simulink model "hamiltonian_record"  (R2012b)
settings: Solver=ode3  StartTime=0.0  StopTime=10  FixedStep=0.001  RelTol=1e-3
settings Model: ExtModeTrigDuration=5000  Creator=yiwei.liu  LastModifiedBy=yiwei.liu
settings SolverCC: PositivePriorityOrder=on
settings RTWCC: SystemTargetFile=quarc_win64.tlc  TemplateMakefile=quarc_default_tmf  Description=QUARC Win64 Target  ProcessScript=quarc_win64_make_rtw_hook
settings STFCustomTargetCC: TargetPreCompLibLocation=C:\PROGRA~3\QUARC\lib\2012b\win64\release  CodeReplacementLibrary=ANSI_C  GeneratePreprocessorConditionals=Disable all  CombineOutputUpdateFcns=on  GRTInterface=off  SystemTargetFile=quarc_win64.tlc
settings GRTTargetCC: TargetPreCompLibLocation=C:\PROGRA~3\QUARC\lib\2012b\win64\release  ParMdlRefBuildCompliant=off  CompOptLevelCompliant=off  ConcurrentExecutionCompliant=off  MatFileLogging=off  ExtMode=on  ExtModeMexFile=quarc_comm

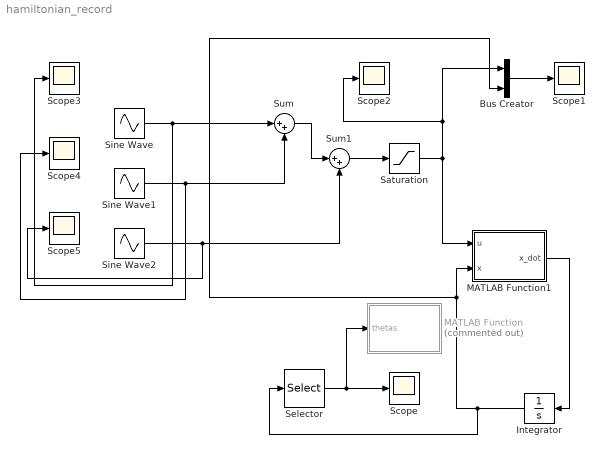
== system hamiltonian_record ==
  Bus Creator : BusCreator  Inputs=2
  Integrator : Integrator  InitialCondition=[0;0;pi;0]
  MATLAB Function : MATLAB Function  Commented=on  TreatAsAtomicUnit=on
  MATLAB Function1 : MATLAB Function  TreatAsAtomicUnit=on
  Saturation : Saturate  UpperLimit=10  LowerLimit=-10
  Scope{,1..5} (6 alike) : Scope
      Scope settings: YMin=-0.25  YMax=5.25
      Scope1 settings: ShowLegends=on  YMin=-7  YMax=8  SaveName=sim  MaxDataPoints=10000
      Scope2 settings: ShowLegends=on  YMin=-7.5  YMax=10  SaveName=rbd1  MaxDataPoints=10000
      Scope3 settings: ShowLegends=on  SaveName=rbd2  MaxDataPoints=10000
      Scope4 settings: ShowLegends=on  SaveName=rbd3  MaxDataPoints=10000
      Scope5 settings: ShowLegends=on  YMin=-3  YMax=7  SaveName=rbd4  MaxDataPoints=10000
  Selector : Selector  InputPortWidth=4  IndexOptions=Index vector (dialog)  Indices=[1 3]  OutputSizes=1
  Sine Wave : Sin  Amplitude=5  Frequency=5  Phase=0.8  SampleTime=0
  Sine Wave1 : Sin  Amplitude=5  Frequency=10  Phase=1.2  SampleTime=0
  Sine Wave2 : Sin  Amplitude=5  Frequency=20  Phase=0.4  SampleTime=0
  Sum : Sum  Inputs=|++
  Sum1 : Sum  Inputs=|++
  wires:
  MATLAB Function1/1(x_dot) -> Integrator/1
  Integrator/1 -> Bus Creator/2, MATLAB Function1/2(x), Selector/1
  Selector/1 -> MATLAB Function/1(thetas), Scope/1
  Sum/1 -> Sum1/1
  Bus Creator/1 -> Scope1/1
  Sine Wave2/1 -> Scope5/1, Sum1/2
  Sine Wave/1 -> Scope3/1, Sum/1
  Sine Wave1/1 -> Scope4/1, Sum/2
  Saturation/1 -> MATLAB Function1/1(u), Scope2/1, Bus Creator/1
  Sum1/1 -> Saturation/1

== matlab function hamiltonian_record/MATLAB Function ==
  data: thetas input
function  fcn(thetas)
%#codegen
A=[0 0 0 0 0];
B=[0 0 6 6 8];
C=[0 -1 -1 0 0];
D=[1 1 1 1 1];

A2=[0 0];
B2=[0 12];
C2=[0 0];
D2=[1 1];
L1=6;

L2=2;
%First Link

    theta1=thetas(1);
    theta2=thetas(2);
    newpoints=trans(theta1,A,B,C,D);
    p= (newpoints(1:1,1:5));

    q= (newpoints(2:2,1:5));

    r= (newpoints(3:3,1:5));
   % Second Link

    new2=trans2(theta2,L1,L2,A2,B2,C2,D2);
    %Frame 1 to frame 0
    x2= new2(1:1,1:2);
    y2= new2(2:2,1:2);
    z2= new2(3:3,1:2);

    new3 = trans(theta1,x2,y2,z2,D2);
    %ABC values of Link 2 in frame 0
    p2= (new3(1:1,1:2));

    q2= (new3(2:2,1:2));

    r2= (new3(3:3,1:2));
   
%     hold on;

    plot3(p,q,r,'-b*',p2,q2,r2,'-g*');
    axis([-15,15,-15,15,-15,15]);
    grid on;
end

== matlab function hamiltonian_record/MATLAB Function1 ==
  data: u input; x_dot output; x input
function x_dot = fcn(u,x)
%#codegen
 
theta1= 0.0304;
theta2= 0.0184;
theta3= 0.0184;
theta4= 0.0921;
theta5= 0.6101;
theta6= 0.0097;

q1 = x(1);
q1_dot = x(2);
q2 = x(3);
q2_dot = x(4);
 
v = [u ; 0];
A = [theta1+theta2*(sin(q2)^2), theta3*cos(q2) ; theta3*cos(q2), theta2];
B = [2*theta2*sin(q2)*cos(q2)*q2_dot, (-1)*theta3*sin(q2)*q2_dot; (-1)*theta2*sin(q2)*cos(q2)*q1_dot,  0];
C = [theta5*q1_dot ; theta6*q2_dot];
D = [0 ;(-1)*theta4*9.8*sin(q2)];
 
%q_dd = [0;0];
q_dd = (A^(-1))*((v - B*[q1_dot ; q2_dot] - C - D)) ;
q1_dd = q_dd(1);
q2_dd = q_dd(2);
x_dot = [q1_dot ;q1_dd ; q2_dot; q2_dd ];
 
end
